simulink model "c2000_host_read_PCMC"  (R2021b)
settings: Solver=FixedStepDiscrete  StartTime=0.0  StopTime=inf  RelTol=1e-3  EnableMultiTasking=on
libraries: instrumentseriallib x3, demo_controls x1, dspstat3 x1
settings Model: Creator=The MathWorks, Inc.  LastModifiedBy=The MathWorks, Inc.
settings SolverCC: AlgebraicLoopSolver=TrustRegion
settings DataIOCC: LimitDataPoints=on  SaveFormat=Array  ReturnWorkspaceOutputs=off
settings OptimizationCC: LifeSpan=1  EfficientTunableParamExpr=on
settings DebuggingCC: UnderspecifiedInitializationDetection=Classic  MergeDetectMultiDrivingBlocksExec=none  SolverPrmCheckMsg=warning  ParameterPrecisionLossMsg=none  AllowSymbolicDim=off  SFUnexpectedBacktrackingDiag=warning  SFNoUnconditionalDefaultTransitionDiag=warning  SFExecutionAtInitializationDiag=none  SFMachineParentedDataDiag=warning  ArithmeticOperatorsInVariantConditions=warning
settings HardwareCC: ProdBitPerPointer=32  ProdBitPerSizeT=32  ProdBitPerPtrDiffT=32  ProdLargestAtomicFloat=None  ProdIntDivRoundTo=Undefined  ProdEndianess=Unspecified  ProdWordSize=32  ProdHWDeviceType=32-bit Generic
settings ModelReferenceCC: PropagateSignalLabelsOutOfModel=off
settings SFSimCC: SimUseLocalCustomCode=off  MATLABDynamicMemAlloc=off  CustomCodeUndefinedFunction=UseInterfaceOnly
settings RTWCC: Description=Real-Time Workshop Embedded Coder  SystemTargetFile=ert.tlc  TemplateMakefile=ert_default_tmf  GenerateReport=on  RTWUseLocalCustomCode=off  IncludeHyperlinkInReport=on  LaunchReport=on  GenerateTraceInfo=on  GenerateTraceReport=on  GenerateTraceReportSl=on  GenerateTraceReportSf=on  GenerateTraceReportEml=on
settings CodeAppCC: IgnoreCustomStorageClasses=off  CustomSymbolStrModelFcn=$N  StateflowObjectComments=on  InternalIdentifier=Classic
settings ERTTargetCC: MultiwordLength=2048  GenerateSampleERTMain=on  ERTCustomFileTemplate=example_file_process.tlc  ConvertIfToSwitch=off  SuppressUnreachableDefaultCases=off
settings ConfigComp: CovMetricSettings=dw  CovSaveCumulativeToWorkspaceVar=on  CovSaveSingleToWorkspaceVar=on  CovExternalEMLEnable=off  CovSFcnEnable=off

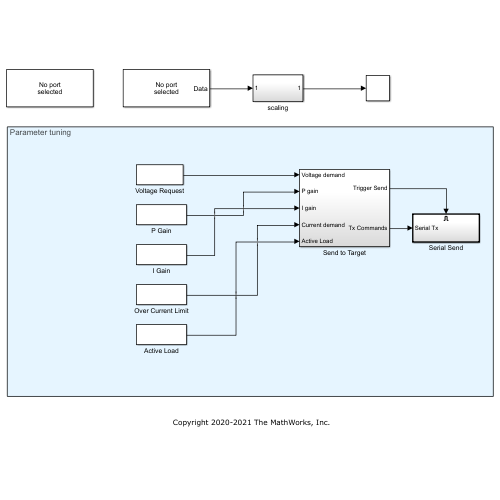
[thumbnail: Simulink's stored preview of the top-level diagram]
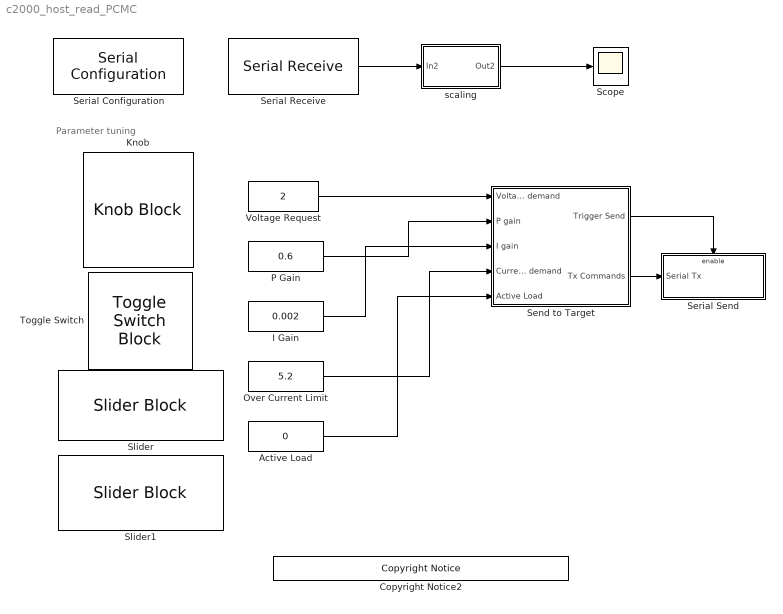
== system c2000_host_read_PCMC ==
  note: Parameter tuning
  Active Load : Constant  Value=0  VectorParams1D=off  OutDataTypeStr=uint16  SampleTime=0.06
  Copyright Notice2 : demo_controls/Copyright Notice  year=2020  prod=tic2000
      settings: SourceProductBaseCode=ME
  I Gain : Constant  Value=0.002  VectorParams1D=off  OutDataTypeStr=single  SampleTime=0.06
  Knob : KnobBlock  ScaleMax=6.99
  Over Current Limit : Constant  Value=5.2  VectorParams1D=off  OutDataTypeStr=single  SampleTime=0.06
  P Gain : Constant  Value=0.6  VectorParams1D=off  OutDataTypeStr=single  SampleTime=0.06
  Scope : Scope
  Send to Target : Subsystem
  Serial Configuration : instrumentseriallib/Serial Configuration  Priority=-200000  Port=<Select a port...>  ComPort=<Select a port...>  BaudRate=6250000  DataBits=8  Parity=none  StopBits=1  ByteOrder=little-endian  FlowControl=none  Timeout=1  SimulateUsing=Interpreted execution  BlockInModel=on
  Serial Receive : instrumentseriallib/Serial Receive  Port=<Select a port...>  ComPort=COM3  DataType=uint16  SaveDataType=uint8  ToggleHeader=on  Header="[ 83  83 ]"  ToggleTerminator=on  Terminator=Custom terminator  CustomTerminator="[ 69  69 ]"  ToggleDataSize=on  DataSize="[1  12000]"  EnableBlockingMode=on  ActionDataUnavailable=Output last received value  ActionWhenDataUnavailable=Output last received value  CustomValue=0  SampleTime=0.06  SimulateUsing=Interpreted execution  BlockInModel=on
  Serial Send : Subsystem  TreatAsAtomicUnit=on
  Slider : SliderBlock  ScaleMax=5.0
  Slider1 : SliderBlock  ScaleMax=2.0
  Toggle Switch : ToggleSwitchBlock
      settings: Values={{'Off', 'On'}, [0 1]}
  Voltage Request : Constant  Value=2  VectorParams1D=off  OutDataTypeStr=single  SampleTime=0.06
  scaling : Subsystem
  wires:
  Voltage Request/1 -> Send to Target/1(Voltage demand)
  P Gain/1 -> Send to Target/2(P gain)
  I Gain/1 -> Send to Target/3(I gain)
  Serial Receive/1 -> scaling/1(In2)
  Send to Target/1(Trigger Send) -> Serial Send/Enable
  Send to Target/2(Tx Commands) -> Serial Send/1(Serial Tx)
  Active Load/1 -> Send to Target/5(Active Load)
  Over Current Limit/1 -> Send to Target/4(Current demand)
  scaling/1(Out2) -> Scope/1

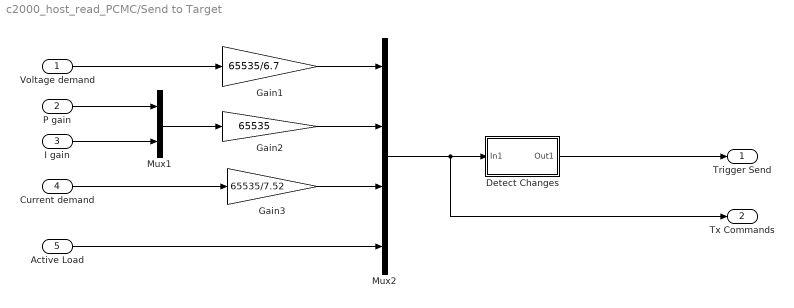
== system c2000_host_read_PCMC/Send to Target ==
  Voltage demand : Inport
  P gain : Inport  Port=2
  I gain : Inport  Port=3
  Current demand : Inport  Port=4
  Active Load : Inport  Port=5
  Detect Changes : Subsystem
  Gain1 : Gain  Gain=65535/6.7  OutDataTypeStr=uint16
  Gain2 : Gain  Gain=65535  OutDataTypeStr=uint16
  Gain3 : Gain  Gain=65535/7.52  OutDataTypeStr=uint16
  Mux1 : Mux  Inputs=2
  Mux2 : Mux
  Trigger Send : Outport  VectorParamsAs1DForOutWhenUnconnected=off
  Tx Commands : Outport  Port=2  VectorParamsAs1DForOutWhenUnconnected=off
  wires:
  Voltage demand/1 -> Gain1/1
  Active Load/1 -> Mux2/4
  P gain/1 -> Mux1/1
  Mux1/1 -> Gain2/1
  Gain2/1 -> Mux2/2
  Mux2/1 -> Tx Commands/1, Detect Changes/1(In1)
  Detect Changes/1(Out1) -> Trigger Send/1
  I gain/1 -> Mux1/2
  Gain1/1 -> Mux2/1
  Current demand/1 -> Gain3/1
  Gain3/1 -> Mux2/3

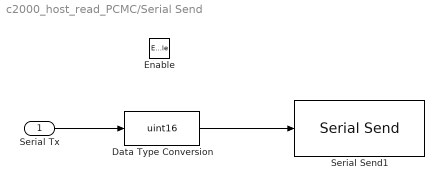
== system c2000_host_read_PCMC/Serial Send ==
  Serial Tx : Inport
  Enable : EnablePort
  Data Type Conversion : DataTypeConversion  OutDataTypeStr=uint16  ConvertRealWorld=Stored Integer (SI)
  Serial Send1 : instrumentseriallib/Serial Send  Port=<Select a port...>  ComPort=COM3  Header=[ 83 ]  Terminator=Custom terminator  CustomTerminator=[ 69 ]  EnableBlockingMode=on  SimulateUsing=Interpreted execution  BlockInModel=on
  wires:
  Data Type Conversion/1 -> Serial Send1/1
  Serial Tx/1 -> Data Type Conversion/1

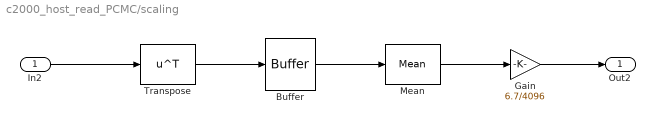
== system c2000_host_read_PCMC/scaling ==
  In2 : Inport
  Buffer : Buffer  N=8  OutputFrames=off
  Gain : Gain  Gain=6.7/4096  OutDataTypeStr=single
  Mean : dspstat3/Mean  run=off  InputProcessing=Columns as channels (frame based)  reset_popup=None  directionMode=Entire input  dimension=8  roiEnable=off  roiType=Rectangles  roiPortion=Entire ROI  roiOutput=Individual statistics for each ROI  roiFlag=off  roundingMode=Floor  overflowMode=off  outputDataTypeStr=Inherit: Same as accumulator  outputMin=[]  outputMax=[]  outputLastDataTypeStr=Inherit: Same as accumulator
  Transpose : Math  Operator=transpose  SignedPower=on  SaturateOnIntegerOverflow=on
  Out2 : Outport  VectorParamsAs1DForOutWhenUnconnected=off
  wires:
  In2/1 -> Transpose/1
  Transpose/1 -> Buffer/1
  Mean/1 -> Gain/1
  Gain/1 -> Out2/1
  Buffer/1 -> Mean/1

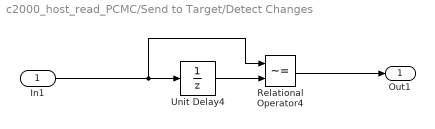
== system c2000_host_read_PCMC/Send to Target/Detect Changes ==
  In1 : Inport
  Relational Operator4 : RelationalOperator  Operator=~=  OutDataTypeStr=boolean  RndMeth=Nearest
  Unit Delay4 : UnitDelay  SampleTime=-1  HasFrameUpgradeWarning=on
  Out1 : Outport  VectorParamsAs1DForOutWhenUnconnected=off
  wires:
  Unit Delay4/1 -> Relational Operator4/2
  In1/1 -> Relational Operator4/1, Unit Delay4/1
  Relational Operator4/1 -> Out1/1
